simulink model "lateral_control_2d"  (R2015a)
settings: Solver=ode45  StartTime=0.0  StopTime=10.0  RelTol=1e-3
undefined symbols (not defined in the file or in its folder): g, HIP_MTR_MAX_CONT_TORQUE, k_sea, kd_lateral, kp_lateral, lateral_offset, lateral_target_angle_right, lateral_transition_force, m_leg, m_leg_motor, m_total_real, max_torque_lateral, maximum_lateral_angle, minimum_lateral_angle
settings Model: Creator=wmartin  LastModifiedBy=wmartin

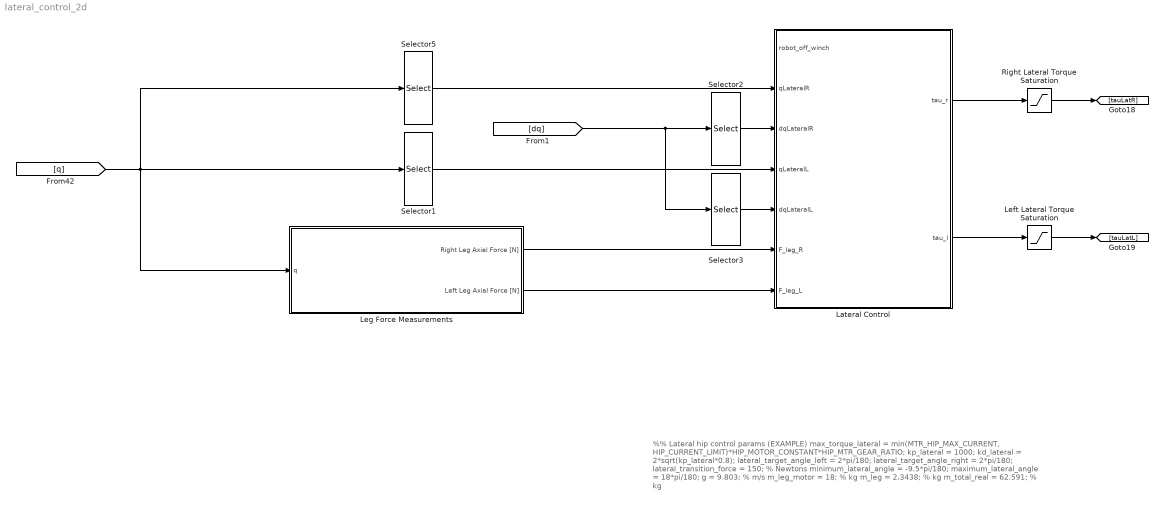
== system lateral_control_2d ==
  note: %% Lateral hip control params (EXAMPLE)
      | max_torque_lateral = min(MTR_HIP_MAX_CURRENT, HIP_CURRENT_LIMIT)*HIP_MOTOR_CONSTANT*HIP_MTR_GEAR_RATIO;
      | kp_lateral = 1000;
      | kd_lateral = 2*sqrt(kp_lateral*0.8);
      | lateral_target_angle_left  =  2*pi/180;
      | lateral_target_angle_right = 2*pi/180;
      | lateral_transition_force = 150; % Newtons
      | minimum_lateral_angle = -9.5*pi/180;
      | maximum_lateral_angle = 18*pi/180;
      |
      | g = 9.803; % m/s
      | m_leg_motor = 18; % kg
      | m_leg = 2.3438; % kg
      | m_total_real = 62.591; % kg
  Lateral Control : MATLAB Function  TreatAsAtomicUnit=on
  Left Lateral Torque Saturation : Saturate  UpperLimit=max_torque_lateral  LowerLimit=-max_torque_lateral
      settings: AttributesFormatString=Top: %<UpperLimit>\nBottom: %<LowerLimit>
  Leg Force Measurements : Subsystem
  Right Lateral Torque Saturation : Saturate  UpperLimit=max_torque_lateral  LowerLimit=-max_torque_lateral
      settings: AttributesFormatString=Top: %<UpperLimit>\nBottom: %<LowerLimit>
  Selector1 : Selector  InputPortWidth=13  Indices=[10]
  Selector2 : Selector  InputPortWidth=13  Indices=[9]
  Selector3 : Selector  InputPortWidth=13  Indices=[10]
  Selector5 : Selector  InputPortWidth=13  Indices=[9]
  wires:
  Lateral Control/1(tau_r) -> Right Lateral Torque Saturation/1
  Right Lateral Torque Saturation/1 -> [tauLatR]
  Left Lateral Torque Saturation/1 -> [tauLatL]
  Lateral Control/2(tau_l) -> Left Lateral Torque Saturation/1
  Leg Force Measurements/1(Right Leg Axial Force [N]) -> Lateral Control/6(F_leg_R)
  Leg Force Measurements/2(Left Leg Axial Force [N]) -> Lateral Control/7(F_leg_L)
  Selector1/1 -> Lateral Control/4(qLateralL)
  Selector5/1 -> Lateral Control/2(qLateralR)
  Selector2/1 -> Lateral Control/3(dqLateralR)
  Selector3/1 -> Lateral Control/5(dqLateralL)
  [q] -> Selector5/1, Leg Force Measurements/1(q), Selector1/1
  ? -> Lateral Control/1(robot_off_winch)
  [dq] -> Selector3/1, Selector2/1

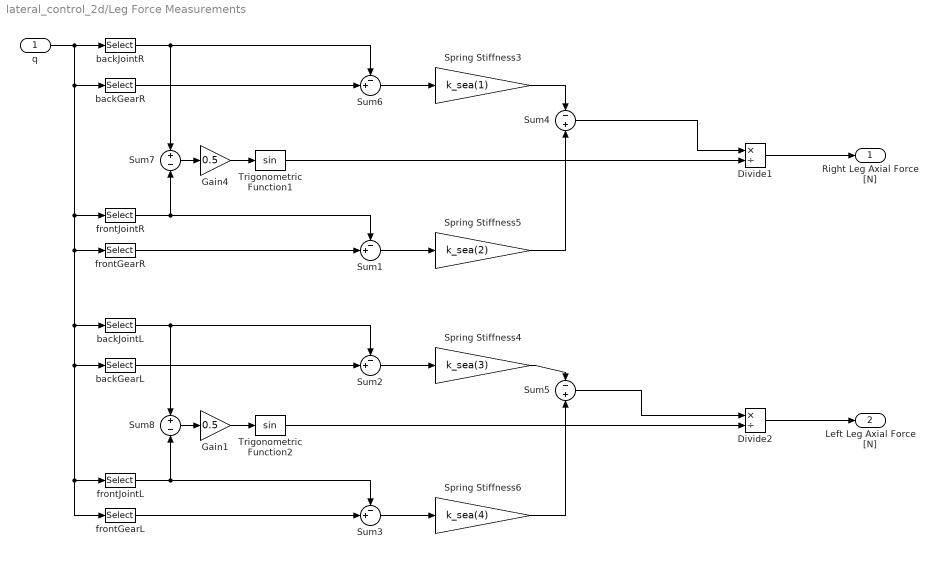
== system lateral_control_2d/Leg Force Measurements ==
  q : Inport
  Divide1 : Product  Inputs=*/
  Divide2 : Product  Inputs=*/
  Gain1 : Gain  Gain=0.5
  Gain4 : Gain  Gain=0.5
  Spring Stiffness3 : Gain  Gain=k_sea(1)
  Spring Stiffness4 : Gain  Gain=k_sea(3)
  Spring Stiffness5 : Gain  Gain=k_sea(2)
  Spring Stiffness6 : Gain  Gain=k_sea(4)
  Sum{1..3,6} (4 alike) : Sum  Inputs=-+|
  Sum4 : Sum  Inputs=-|+
  Sum5 : Sum  Inputs=-|+
  Sum7 : Sum  Inputs=+|-
  Sum8 : Sum  Inputs=+|-
  Trigonometric Function1 : Trigonometry
  Trigonometric Function2 : Trigonometry
  backGearL : Selector  InputPortWidth=13  Indices=[6]
  backGearR : Selector  InputPortWidth=13  Indices=[2]
  backJointL : Selector  InputPortWidth=13  Indices=[5]
  backJointR : Selector  InputPortWidth=13  Indices=[1]
  frontGearL : Selector  InputPortWidth=13  Indices=[8]
  frontGearR : Selector  InputPortWidth=13  Indices=[4]
  frontJointL : Selector  InputPortWidth=13  Indices=[7]
  frontJointR : Selector  InputPortWidth=13  Indices=[3]
  Right Leg Axial Force [N] : Outport
  Left Leg Axial Force [N] : Outport  Port=2
  wires:
  Sum3/1 -> Spring Stiffness6/1
  Sum2/1 -> Spring Stiffness4/1
  backJointL/1 -> Sum8/1, Sum2/1
  frontGearL/1 -> Sum3/2
  frontJointL/1 -> Sum8/2, Sum3/1
  backGearL/1 -> Sum2/2
  Sum6/1 -> Spring Stiffness3/1
  Sum1/1 -> Spring Stiffness5/1
  backJointR/1 -> Sum6/1, Sum7/1
  frontGearR/1 -> Sum1/2
  frontJointR/1 -> Sum1/1, Sum7/2
  backGearR/1 -> Sum6/2
  q/1 -> backGearR/1, frontJointR/1, backJointL/1, frontJointL/1, frontGearL/1, backGearL/1, frontGearR/1, backJointR/1
  Spring Stiffness3/1 -> Sum4/1
  Spring Stiffness5/1 -> Sum4/2
  Spring Stiffness6/1 -> Sum5/2
  Sum4/1 -> Divide1/1
  Sum5/1 -> Divide2/1
  Trigonometric Function1/1 -> Divide1/2
  Trigonometric Function2/1 -> Divide2/2
  Divide1/1 -> Right Leg Axial Force [N]/1
  Divide2/1 -> Left Leg Axial Force [N]/1
  Spring Stiffness4/1 -> Sum5/1
  Sum7/1 -> Gain4/1
  Gain4/1 -> Trigonometric Function1/1
  Gain1/1 -> Trigonometric Function2/1
  Sum8/1 -> Gain1/1

== matlab function lateral_control_2d/Lateral Control ==
  data: robot_off_winch input; tau_r output size=1; qLateralR input; dqLateralR input; qLateralL input; dqLateralL input; F_leg_R input; F_leg_L input; lateral_transition_force parameter; lateral_target_angle_right parameter; m_leg_motor parameter; m_leg parameter; m_total_real parameter; g parameter; lateral_offset parameter; tau_l output size=1; kp_lateral parameter; kd_lateral parameter; minimum_lateral_angle parameter; maximum_lateral_angle parameter; HIP_MTR_MAX_CONT_TORQUE parameter
function [tau_r, tau_l] = LateralBoomControl(robot_off_winch, qLateralR, dqLateralR, qLateralL, dqLateralL, F_leg_R, F_leg_L, lateral_transition_force, lateral_target_angle_right, m_leg_motor, m_leg, m_total_real, g, lateral_offset, kp_lateral, kd_lateral, minimum_lateral_angle, maximum_lateral_angle, HIP_MTR_MAX_CONT_TORQUE)
    
    % Only add gravity compensation to PD when suspended from winch (approximately static)
    gravity_compensation = 0;
    if ~robot_off_winch, gravity_compensation = (m_leg_motor+m_leg)*g*lateral_offset; end
    
    % Inertia for feedforward accelerations
    motor_inertia = (m_leg_motor+m_leg)*lateral_offset^2;
    
    % Right Leg
    right_target = [lateral_target_angle_right, 0, 0];
    desired = [saturate(right_target(1),minimum_lateral_angle,maximum_lateral_angle), right_target(2)];
    measured = [qLateralR, dqLateralR];
    tau_r = [kp_lateral, kd_lateral] * (desired-measured)' + gravity_compensation + motor_inertia*right_target(3);
    tau_r = max(min(HIP_MTR_MAX_CONT_TORQUE, tau_r),-HIP_MTR_MAX_CONT_TORQUE);
    
    if (F_leg_R >= lateral_transition_force)
        if robot_off_winch
            tau_r = -F_leg_R*lateral_offset*(m_total_real-(m_leg_motor+m_leg))/m_total_real;
        else
            tau_r = -lateral_offset*(F_leg_R-(m_leg_motor+m_leg)*g);
        end
    end
    
    % Left Leg
    left_target = [lateral_target_angle_right, 0, 0];
    desired = [saturate(left_target(1),minimum_lateral_angle,maximum_lateral_angle), left_target(2)];
    measured = [qLateralL, dqLateralL];
    tau_l = [kp_lateral, kd_lateral] * (desired-measured)' + gravity_compensation + motor_inertia*left_target(3);
    tau_l = max(min(HIP_MTR_MAX_CONT_TORQUE, tau_l),-HIP_MTR_MAX_CONT_TORQUE);
    
    if (F_leg_L >= lateral_transition_force)
        if robot_off_winch
            tau_l = -F_leg_L*lateral_offset*(m_total_real-(m_leg_motor+m_leg))/m_total_real;
        else
            tau_l = -lateral_offset*(F_leg_L-(m_leg_motor+m_leg)*g);
        end
    end
end

function [desired_saturated] = saturate(desired, minimum_lateral_angle, maximum_lateral_angle)
    desired_saturated = desired;
    if desired(1) < minimum_lateral_angle
        desired_saturated = [minimum_lateral_angle, 0];
    elseif desired(1) > maximum_lateral_angle
        desired_saturated = [maximum_lateral_angle, 0];    
    end
end
